simulink model "Week3_prob3"  (R2020b)
settings: Solver=VariableStepAuto  StartTime=0.0  StopTime=20.0  RelTol=1e-3
values from neighbouring files (symbols this model uses):
  g = 9.81    [week3_project3.sldd]
  J = 0.01    [week3_project3.sldd]
  K = 1000.0    [week3_project3.sldd]
  m = 1200.0    [week3_project3.sldd]
  R = 0.28    [week3_project3.sldd]
  T = 0.01    [week3_project3.sldd]
  Tbmax = 2000.0    [week3_project3.sldd]
  Vmin = 1.4    [week3_project3.sldd]
settings Model: DataDictionary=week3_project3.sldd  Creator=user  LastModifiedBy=user

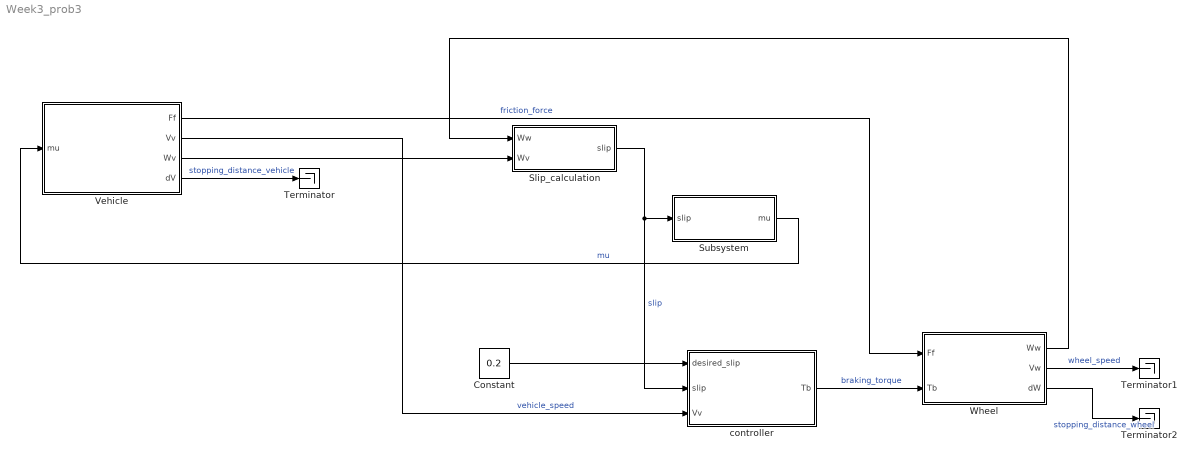
== system Week3_prob3 ==
  Constant : Constant  Value=0.2
  Slip_calculation : Subsystem
  Subsystem : Subsystem
  Terminator : Terminator
  Terminator1 : Terminator
  Terminator2 : Terminator
  Vehicle : Subsystem
  Wheel : Subsystem
  controller : Subsystem
  wires:
  Vehicle/2(Vv) -> controller/3(Vv)  "vehicle_speed"
  Vehicle/3(Wv) -> Slip_calculation/2(Wv)
  controller/1(Tb) -> Wheel/2(Tb)  "braking_torque"
  Subsystem/1(mu) -> Vehicle/1(mu)  "mu"
  Vehicle/1(Ff) -> Wheel/1(Ff)  "friction_force"
  Wheel/1(Ww) -> Slip_calculation/1(Ww)
  Vehicle/4(dV) -> Terminator/1  "stopping_distance_vehicle"
  Wheel/2(Vw) -> Terminator1/1  "wheel_speed"
  Slip_calculation/1(slip) -> controller/2(slip), Subsystem/1(slip)  "slip"
  Wheel/3(dW) -> Terminator2/1  "stopping_distance_wheel"
  Constant/1 -> controller/1(desired_slip)

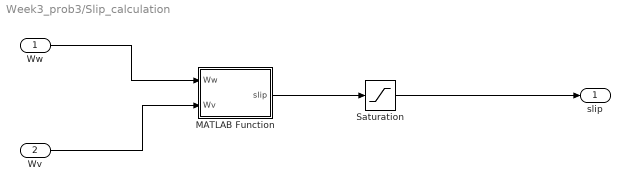
== system Week3_prob3/Slip_calculation ==
  Ww : Inport
  Wv : Inport  Port=2
  MATLAB Function : MATLAB Function  TreatAsAtomicUnit=on
  Saturation : Saturate  UpperLimit=1  LowerLimit=0
  slip : Outport
  wires:
  Ww/1 -> MATLAB Function/1(Ww)
  Wv/1 -> MATLAB Function/2(Wv)
  MATLAB Function/1(slip) -> Saturation/1
  Saturation/1 -> slip/1

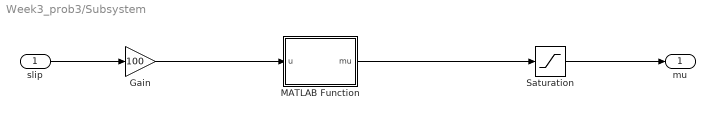
== system Week3_prob3/Subsystem ==
  slip : Inport
  Gain : Gain  Gain=100
  MATLAB Function : MATLAB Function  TreatAsAtomicUnit=on
  Saturation : Saturate  UpperLimit=1  LowerLimit=0
  mu : Outport
  wires:
  Saturation/1 -> mu/1
  slip/1 -> Gain/1
  Gain/1 -> MATLAB Function/1(u)
  MATLAB Function/1(mu) -> Saturation/1

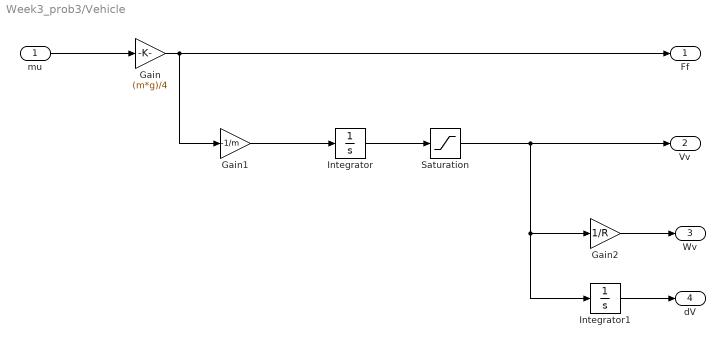
== system Week3_prob3/Vehicle ==
  mu : Inport
  Gain : Gain  Gain=(m*g)/4
  Gain1 : Gain  Gain=-1/m
  Gain2 : Gain  Gain=1/R
  Integrator : Integrator  InitialCondition=28
  Integrator1 : Integrator
  Saturation : Saturate  UpperLimit=1000  LowerLimit=0.001
  Ff : Outport
  Vv : Outport  Port=2
  Wv : Outport  Port=3
  dV : Outport  Port=4
  wires:
  mu/1 -> Gain/1
  Gain/1 -> Gain1/1, Ff/1
  Gain1/1 -> Integrator/1
  Integrator/1 -> Saturation/1
  Saturation/1 -> Integrator1/1, Gain2/1, Vv/1
  Gain2/1 -> Wv/1
  Integrator1/1 -> dV/1

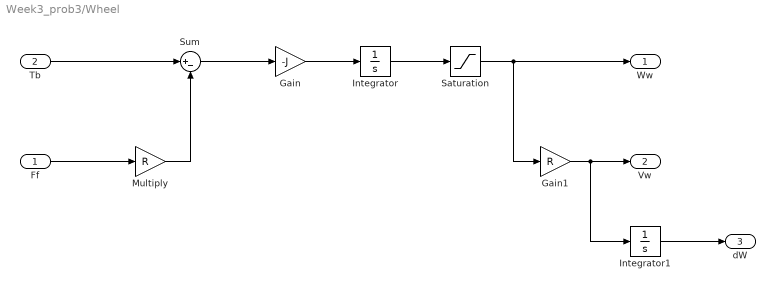
== system Week3_prob3/Wheel ==
  Ff : Inport
  Tb : Inport  Port=2
  Gain : Gain  Gain=-J
  Gain1 : Gain  Gain=R
  Integrator : Integrator  InitialCondition=28/R
  Integrator1 : Integrator
  Multiply : Gain  Gain=R
  Saturation : Saturate  UpperLimit=1000  LowerLimit=0
  Sum : Sum  Inputs=|+-
  Ww : Outport
  Vw : Outport  Port=2
  dW : Outport  Port=3
  wires:
  Ff/1 -> Multiply/1
  Tb/1 -> Sum/1
  Multiply/1 -> Sum/2
  Sum/1 -> Gain/1
  Gain/1 -> Integrator/1
  Integrator/1 -> Saturation/1
  Saturation/1 -> Gain1/1, Ww/1
  Gain1/1 -> Integrator1/1, Vw/1
  Integrator1/1 -> dW/1

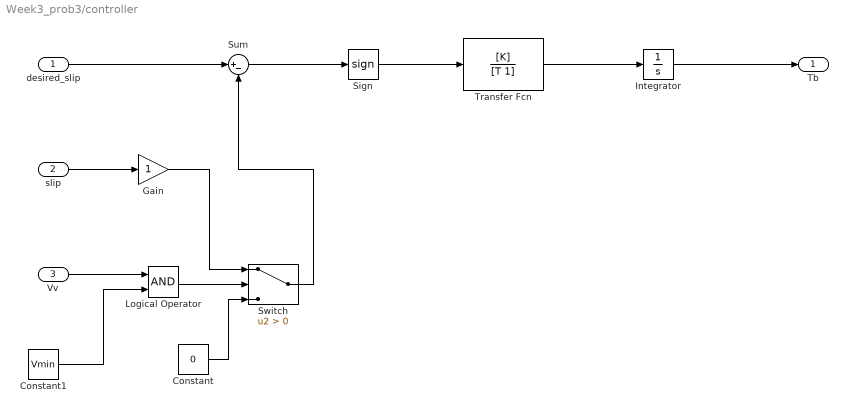
== system Week3_prob3/controller ==
  desired_slip : Inport
  slip : Inport  Port=2
  Vv : Inport  Port=3
  Constant : Constant  Value=0
  Constant1 : Constant  Value=Vmin
  Gain : Gain
  Integrator : Integrator  LimitOutput=on  UpperSaturationLimit=Tbmax  LowerSaturationLimit=0
  Logical Operator : Logic  AllPortsSameDT=off  OutDataTypeStr=boolean
  Sign : Signum
  Sum : Sum  Inputs=|+-
  Switch : Switch  Criteria=u2 > Threshold
  Transfer Fcn : TransferFcn  Numerator=[K]  Denominator=[T 1]
  Tb : Outport
  wires:
  slip/1 -> Gain/1
  Vv/1 -> Logical Operator/1
  Logical Operator/1 -> Switch/2
  Integrator/1 -> Tb/1
  desired_slip/1 -> Sum/1
  Switch/1 -> Sum/2
  Constant/1 -> Switch/3
  Constant1/1 -> Logical Operator/2
  Gain/1 -> Switch/1
  Sum/1 -> Sign/1
  Sign/1 -> Transfer Fcn/1
  Transfer Fcn/1 -> Integrator/1

== matlab function Week3_prob3/Slip_calculation/MATLAB Function ==
  data: Ww input; slip output; Wv input
function slip = fcn(Ww, Wv)

slip=1-(Ww/(Wv+(Wv==0)*eps));

== matlab function Week3_prob3/Subsystem/MATLAB Function ==
  data: u input; mu output
function mu = fcn(u)

mu=0.7*(1.07*(1-exp(-0.5*u)-0.003*u));
